simulink model "simVehicle"  (R2016a)
settings: Solver=FixedStepDiscrete  StartTime=0.0  StopTime=1000000000  FixedStep=0.1  RelTol=1e-3
libraries: simulink x6
settings Model: Creator=Brian Jackson  LastModifiedBy=Brian Jackson

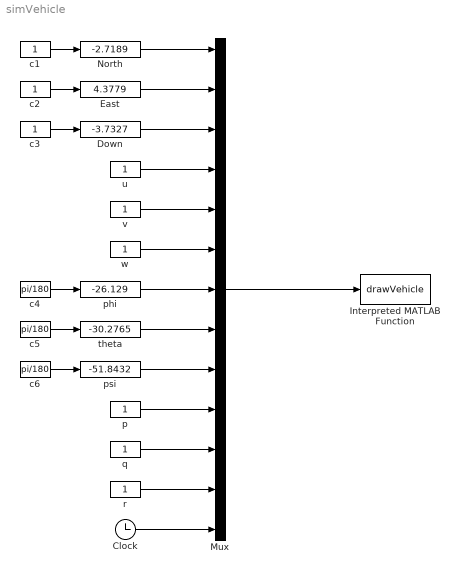
== system simVehicle ==
  Clock : Clock
  Down : simulink/Math Operations/Slider Gain  low=-10  gain=-3.7327  high=10
  East : simulink/Math Operations/Slider Gain  low=-10  gain=4.3779  high=10
  Interpreted MATLAB Function : MATLABFcn  MATLABFcn=drawVehicle  OutputDimensions=0
  Mux : Mux  Inputs=13
  North : simulink/Math Operations/Slider Gain  low=-10  gain=-2.7189  high=10
  c1 : Constant
  c2 : Constant
  c3 : Constant
  c4 : Constant  Value=pi/180
  c5 : Constant  Value=pi/180
  c6 : Constant  Value=pi/180
  p : Constant
  phi : simulink/Math Operations/Slider Gain  low=-90  gain=-26.129  high=90
  psi : simulink/Math Operations/Slider Gain  low=-90  gain=-51.8432  high=90
  q : Constant
  r : Constant
  theta : simulink/Math Operations/Slider Gain  low=-90  gain=-30.2765  high=90
  u : Constant
  v : Constant
  w : Constant
  wires:
  North/1 -> Mux/1
  East/1 -> Mux/2
  Down/1 -> Mux/3
  u/1 -> Mux/4
  v/1 -> Mux/5
  w/1 -> Mux/6
  phi/1 -> Mux/7
  theta/1 -> Mux/8
  psi/1 -> Mux/9
  p/1 -> Mux/10
  q/1 -> Mux/11
  r/1 -> Mux/12
  Clock/1 -> Mux/13
  c2/1 -> East/1
  c3/1 -> Down/1
  c1/1 -> North/1
  c4/1 -> phi/1
  c5/1 -> theta/1
  c6/1 -> psi/1
  Mux/1 -> Interpreted MATLAB Function/1
